simulink model "GPCA_Alarm"  (Simulink 8.7)
settings: Solver=VariableStepAuto  StartTime=0.0  StopTime=10.0  RelTol=1e-3
libraries: simulink x14
(part 2 of 3)

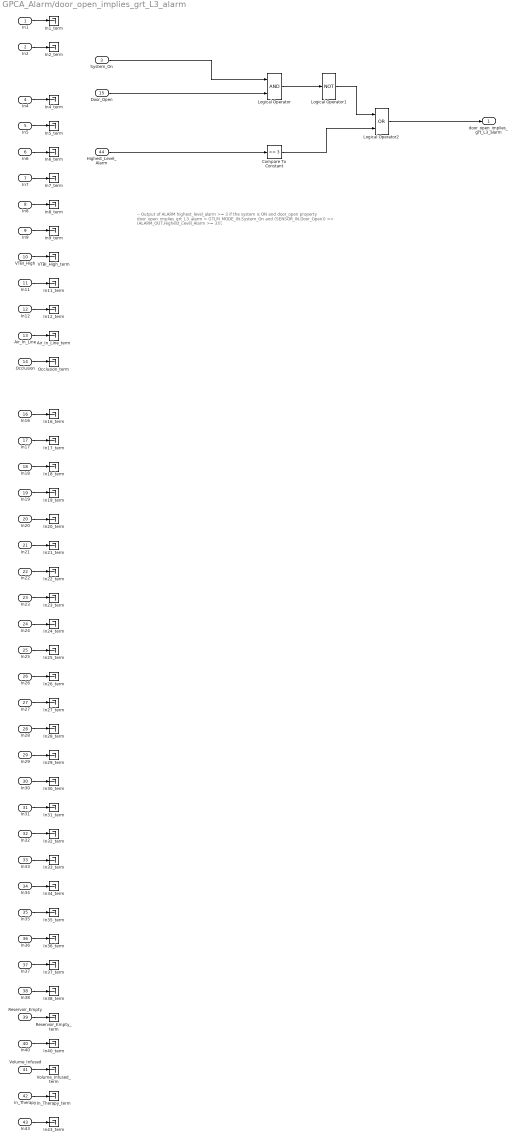
== system GPCA_Alarm/door_open_implies_grt_L3_alarm ==
  note: -- Output of ALARM highest_level_alarm >= 3 if the system is ON and door_open
      | property door_open_implies_grt_L3_alarm =
      | ((TLM_MODE_IN.System_On and (SENSOR_IN.Door_Open)) => (ALARM_OUT.Highest_Level_Alarm >= 3));
  In1 : Inport
  In2 : Inport  Port=2
  System_On : Inport  Port=3
  In4 : Inport  Port=4
  In5 : Inport  Port=5
  In6 : Inport  Port=6
  In7 : Inport  Port=7
  In8 : Inport  Port=8
  In9 : Inport  Port=9
  VTBI_High : Inport  Port=10
  In11 : Inport  Port=11
  In12 : Inport  Port=12
  Air_In_Line : Inport  Port=13
  Occlusion : Inport  Port=14
  Door_Open : Inport  Port=15
  In16 : Inport  Port=16
  In17 : Inport  Port=17
  In18 : Inport  Port=18
  In19 : Inport  Port=19
  In20 : Inport  Port=20
  In21 : Inport  Port=21
  In22 : Inport  Port=22
  In23 : Inport  Port=23
  In24 : Inport  Port=24
  In25 : Inport  Port=25
  In26 : Inport  Port=26
  In27 : Inport  Port=27
  In28 : Inport  Port=28
  In29 : Inport  Port=29
  In30 : Inport  Port=30
  In31 : Inport  Port=31
  In32 : Inport  Port=32
  In33 : Inport  Port=33
  In34 : Inport  Port=34
  In35 : Inport  Port=35
  In36 : Inport  Port=36
  In37 : Inport  Port=37
  In38 : Inport  Port=38
  Reservoir_Empty : Inport  Port=39
  In40 : Inport  Port=40
  Volume_Infused : Inport  Port=41
  In_Therapy : Inport  Port=42
  In43 : Inport  Port=43
  Highest_Level_Alarm : Inport  Port=44
  Air_In_Line_term : Terminator
  Compare To Constant : simulink/Logic and Bit Operations/Compare To Constant  relop=>=  const=3  OutDataTypeStr=boolean
  In11_term : Terminator
  In12_term : Terminator
  In16_term : Terminator
  In17_term : Terminator
  In18_term : Terminator
  In19_term : Terminator
  In1_term : Terminator
  In20_term : Terminator
  In21_term : Terminator
  In22_term : Terminator
  In23_term : Terminator
  In24_term : Terminator
  In25_term : Terminator
  In26_term : Terminator
  In27_term : Terminator
  In28_term : Terminator
  In29_term : Terminator
  In2_term : Terminator
  In30_term : Terminator
  In31_term : Terminator
  In32_term : Terminator
  In33_term : Terminator
  In34_term : Terminator
  In35_term : Terminator
  In36_term : Terminator
  In37_term : Terminator
  In38_term : Terminator
  In40_term : Terminator
  In43_term : Terminator
  In4_term : Terminator
  In5_term : Terminator
  In6_term : Terminator
  In7_term : Terminator
  In8_term : Terminator
  In9_term : Terminator
  In_Therapy_term : Terminator
  Logical Operator : Logic  AllPortsSameDT=off  OutDataTypeStr=boolean
  Logical Operator1 : Logic  Operator=NOT  Inputs=3  AllPortsSameDT=off  OutDataTypeStr=boolean
  Logical Operator2 : Logic  Operator=OR  AllPortsSameDT=off  OutDataTypeStr=boolean
  Occlusion_term : Terminator
  Reservoir_Empty_term : Terminator
  VTBI_High_term : Terminator
  Volume_Infused_term : Terminator
  door_open_implies_grt_L3_alarm : Outport
  wires:
  In1/1 -> In1_term/1
  In2/1 -> In2_term/1
  In4/1 -> In4_term/1
  In5/1 -> In5_term/1
  In6/1 -> In6_term/1
  In7/1 -> In7_term/1
  In8/1 -> In8_term/1
  In9/1 -> In9_term/1
  VTBI_High/1 -> VTBI_High_term/1
  In11/1 -> In11_term/1
  In12/1 -> In12_term/1
  Air_In_Line/1 -> Air_In_Line_term/1
  Occlusion/1 -> Occlusion_term/1
  In16/1 -> In16_term/1
  In17/1 -> In17_term/1
  In18/1 -> In18_term/1
  In19/1 -> In19_term/1
  In20/1 -> In20_term/1
  In21/1 -> In21_term/1
  In22/1 -> In22_term/1
  In23/1 -> In23_term/1
  In24/1 -> In24_term/1
  In25/1 -> In25_term/1
  In26/1 -> In26_term/1
  In27/1 -> In27_term/1
  In28/1 -> In28_term/1
  In29/1 -> In29_term/1
  In30/1 -> In30_term/1
  In31/1 -> In31_term/1
  In32/1 -> In32_term/1
  In33/1 -> In33_term/1
  In34/1 -> In34_term/1
  In35/1 -> In35_term/1
  In36/1 -> In36_term/1
  In37/1 -> In37_term/1
  In38/1 -> In38_term/1
  Reservoir_Empty/1 -> Reservoir_Empty_term/1
  In40/1 -> In40_term/1
  Volume_Infused/1 -> Volume_Infused_term/1
  In_Therapy/1 -> In_Therapy_term/1
  In43/1 -> In43_term/1
  System_On/1 -> Logical Operator/1
  Door_Open/1 -> Logical Operator/2
  Highest_Level_Alarm/1 -> Compare To Constant/1
  Logical Operator/1 -> Logical Operator1/1
  Logical Operator1/1 -> Logical Operator2/1
  Compare To Constant/1 -> Logical Operator2/2
  Logical Operator2/1 -> door_open_implies_grt_L3_alarm/1

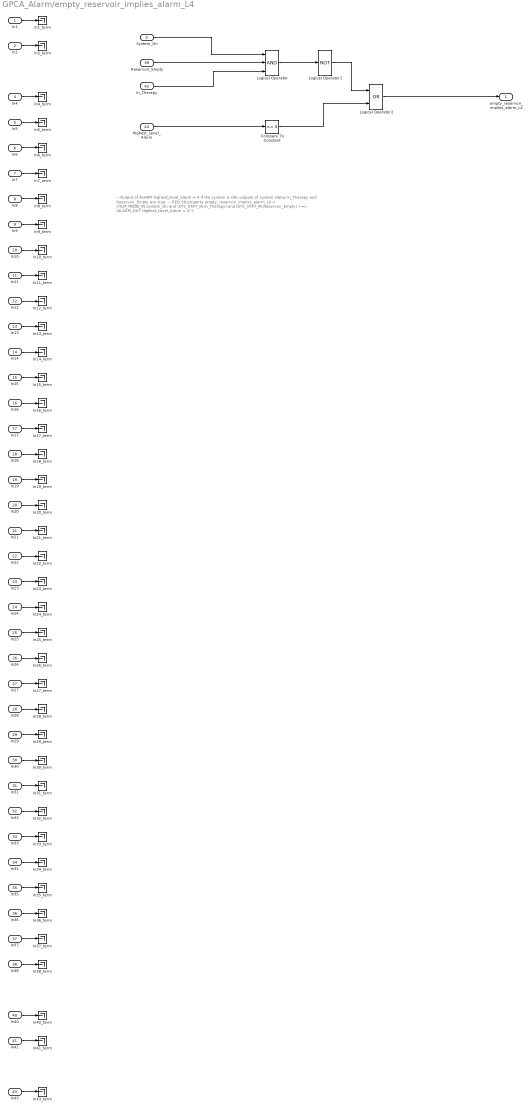
== system GPCA_Alarm/empty_reservoir_implies_alarm_L4 ==
  note: -- Output of ALARM highest_level_alarm = 4 if the system is ON, outputs of system status In_Therapy and Reservoir_Empty are true.
      | -- REQ 59
      | property empty_reservoir_implies_alarm_L4 =
      | ((TLM_MODE_IN.System_On and (SYS_STAT_IN.In_Therapy) and (SYS_STAT_IN.Reservoir_Empty) ) =>
      | (ALARM_OUT.Highest_Level_Alarm = 4) );
  In1 : Inport
  In2 : Inport  Port=2
  System_On : Inport  Port=3
  In4 : Inport  Port=4
  In5 : Inport  Port=5
  In6 : Inport  Port=6
  In7 : Inport  Port=7
  In8 : Inport  Port=8
  In9 : Inport  Port=9
  In10 : Inport  Port=10
  In11 : Inport  Port=11
  In12 : Inport  Port=12
  In13 : Inport  Port=13
  In14 : Inport  Port=14
  In15 : Inport  Port=15
  In16 : Inport  Port=16
  In17 : Inport  Port=17
  In18 : Inport  Port=18
  In19 : Inport  Port=19
  In20 : Inport  Port=20
  In21 : Inport  Port=21
  In22 : Inport  Port=22
  In23 : Inport  Port=23
  In24 : Inport  Port=24
  In25 : Inport  Port=25
  In26 : Inport  Port=26
  In27 : Inport  Port=27
  In28 : Inport  Port=28
  In29 : Inport  Port=29
  In30 : Inport  Port=30
  In31 : Inport  Port=31
  In32 : Inport  Port=32
  In33 : Inport  Port=33
  In34 : Inport  Port=34
  In35 : Inport  Port=35
  In36 : Inport  Port=36
  In37 : Inport  Port=37
  In38 : Inport  Port=38
  Reservoir_Empty : Inport  Port=39
  In40 : Inport  Port=40
  In41 : Inport  Port=41
  In_Therapy : Inport  Port=42
  In43 : Inport  Port=43
  Highest_Level_Alarm : Inport  Port=44
  Compare To Constant : simulink/Logic and Bit Operations/Compare To Constant  relop===  const=4  OutDataTypeStr=boolean
  In10_term : Terminator
  In11_term : Terminator
  In12_term : Terminator
  In13_term : Terminator
  In14_term : Terminator
  In15_term : Terminator
  In16_term : Terminator
  In17_term : Terminator
  In18_term : Terminator
  In19_term : Terminator
  In1_term : Terminator
  In20_term : Terminator
  In21_term : Terminator
  In22_term : Terminator
  In23_term : Terminator
  In24_term : Terminator
  In25_term : Terminator
  In26_term : Terminator
  In27_term : Terminator
  In28_term : Terminator
  In29_term : Terminator
  In2_term : Terminator
  In30_term : Terminator
  In31_term : Terminator
  In32_term : Terminator
  In33_term : Terminator
  In34_term : Terminator
  In35_term : Terminator
  In36_term : Terminator
  In37_term : Terminator
  In38_term : Terminator
  In40_term : Terminator
  In41_term : Terminator
  In43_term : Terminator
  In4_term : Terminator
  In5_term : Terminator
  In6_term : Terminator
  In7_term : Terminator
  In8_term : Terminator
  In9_term : Terminator
  Logical Operator : Logic  Inputs=3  AllPortsSameDT=off  OutDataTypeStr=boolean
  Logical Operator1 : Logic  Operator=NOT  Inputs=3  AllPortsSameDT=off  OutDataTypeStr=boolean
  Logical Operator2 : Logic  Operator=OR  AllPortsSameDT=off  OutDataTypeStr=boolean
  empty_reservoir_implies_alarm_L4 : Outport
  wires:
  In1/1 -> In1_term/1
  In2/1 -> In2_term/1
  System_On/1 -> Logical Operator/1
  In4/1 -> In4_term/1
  In5/1 -> In5_term/1
  In6/1 -> In6_term/1
  In7/1 -> In7_term/1
  In8/1 -> In8_term/1
  In9/1 -> In9_term/1
  In10/1 -> In10_term/1
  In11/1 -> In11_term/1
  In12/1 -> In12_term/1
  In13/1 -> In13_term/1
  In14/1 -> In14_term/1
  In15/1 -> In15_term/1
  In16/1 -> In16_term/1
  In17/1 -> In17_term/1
  In18/1 -> In18_term/1
  In19/1 -> In19_term/1
  In20/1 -> In20_term/1
  In21/1 -> In21_term/1
  In22/1 -> In22_term/1
  In23/1 -> In23_term/1
  In24/1 -> In24_term/1
  In25/1 -> In25_term/1
  In26/1 -> In26_term/1
  In27/1 -> In27_term/1
  In28/1 -> In28_term/1
  In29/1 -> In29_term/1
  In30/1 -> In30_term/1
  In31/1 -> In31_term/1
  In32/1 -> In32_term/1
  In33/1 -> In33_term/1
  In34/1 -> In34_term/1
  In35/1 -> In35_term/1
  In36/1 -> In36_term/1
  In37/1 -> In37_term/1
  In38/1 -> In38_term/1
  Reservoir_Empty/1 -> Logical Operator/2
  In40/1 -> In40_term/1
  In41/1 -> In41_term/1
  In_Therapy/1 -> Logical Operator/3
  In43/1 -> In43_term/1
  Highest_Level_Alarm/1 -> Compare To Constant/1
  Logical Operator/1 -> Logical Operator1/1
  Logical Operator1/1 -> Logical Operator2/1
  Compare To Constant/1 -> Logical Operator2/2
  Logical Operator2/1 -> empty_reservoir_implies_alarm_L4/1

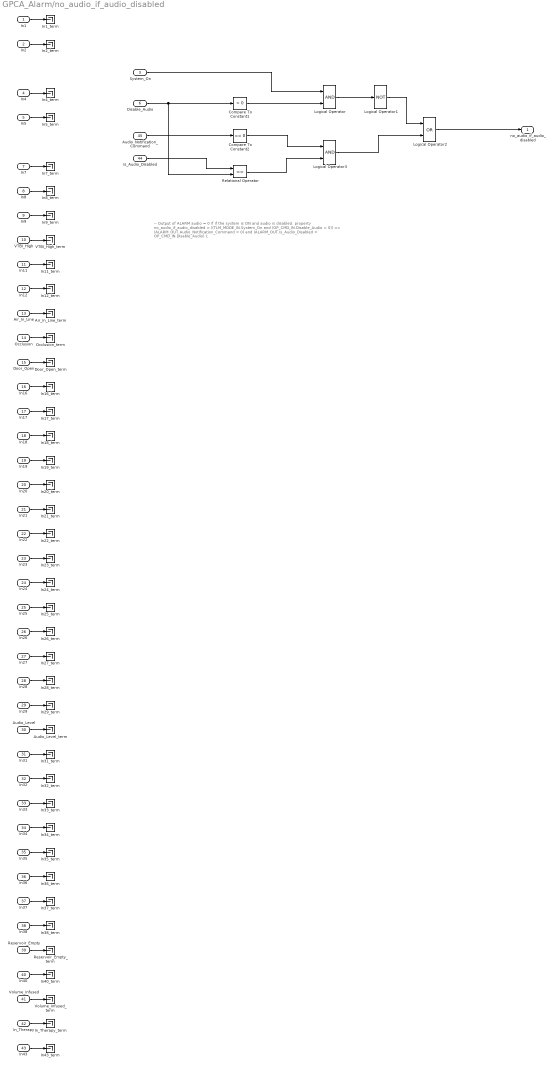
== system GPCA_Alarm/no_audio_if_audio_disabled ==
  note: -- Output of ALARM audio = 0 if if the system is ON and audio is disabled.
      | property no_audio_if_audio_disabled =
      | ((TLM_MODE_IN.System_On and (OP_CMD_IN.Disable_Audio > 0))
      | => (ALARM_OUT.Audio_Notification_Command = 0) and (ALARM_OUT.Is_Audio_Disabled = OP_CMD_IN.Disable_Audio) );
  In1 : Inport
  In2 : Inport  Port=2
  System_On : Inport  Port=3
  In4 : Inport  Port=4
  In5 : Inport  Port=5
  Disable_Audio : Inport  Port=6
  In7 : Inport  Port=7
  In8 : Inport  Port=8
  In9 : Inport  Port=9
  VTBI_High : Inport  Port=10
  In11 : Inport  Port=11
  In12 : Inport  Port=12
  Air_In_Line : Inport  Port=13
  Occlusion : Inport  Port=14
  Door_Open : Inport  Port=15
  In16 : Inport  Port=16
  In17 : Inport  Port=17
  In18 : Inport  Port=18
  In19 : Inport  Port=19
  In20 : Inport  Port=20
  In21 : Inport  Port=21
  In22 : Inport  Port=22
  In23 : Inport  Port=23
  In24 : Inport  Port=24
  In25 : Inport  Port=25
  In26 : Inport  Port=26
  In27 : Inport  Port=27
  In28 : Inport  Port=28
  In29 : Inport  Port=29
  Audio_Level : Inport  Port=30
  In31 : Inport  Port=31
  In32 : Inport  Port=32
  In33 : Inport  Port=33
  In34 : Inport  Port=34
  In35 : Inport  Port=35
  In36 : Inport  Port=36
  In37 : Inport  Port=37
  In38 : Inport  Port=38
  Reservoir_Empty : Inport  Port=39
  In40 : Inport  Port=40
  Volume_Infused : Inport  Port=41
  In_Therapy : Inport  Port=42
  In43 : Inport  Port=43
  Is_Audio_Disabled : Inport  Port=44
  Audio_Notification_Command : Inport  Port=45
  Air_In_Line_term : Terminator
  Audio_Level_term : Terminator
  Compare To Constant1 : simulink/Logic and Bit Operations/Compare To Constant  relop=>  const=0  OutDataTypeStr=boolean
  Compare To Constant2 : simulink/Logic and Bit Operations/Compare To Constant  relop===  const=0  OutDataTypeStr=boolean
  Door_Open_term : Terminator
  In11_term : Terminator
  In12_term : Terminator
  In16_term : Terminator
  In17_term : Terminator
  In18_term : Terminator
  In19_term : Terminator
  In1_term : Terminator
  In20_term : Terminator
  In21_term : Terminator
  In22_term : Terminator
  In23_term : Terminator
  In24_term : Terminator
  In25_term : Terminator
  In26_term : Terminator
  In27_term : Terminator
  In28_term : Terminator
  In29_term : Terminator
  In2_term : Terminator
  In31_term : Terminator
  In32_term : Terminator
  In33_term : Terminator
  In34_term : Terminator
  In35_term : Terminator
  In36_term : Terminator
  In37_term : Terminator
  In38_term : Terminator
  In40_term : Terminator
  In43_term : Terminator
  In4_term : Terminator
  In5_term : Terminator
  In7_term : Terminator
  In8_term : Terminator
  In9_term : Terminator
  In_Therapy_term : Terminator
  Logical Operator : Logic  AllPortsSameDT=off  OutDataTypeStr=boolean
  Logical Operator1 : Logic  Operator=NOT  Inputs=3  AllPortsSameDT=off  OutDataTypeStr=boolean
  Logical Operator2 : Logic  Operator=OR  AllPortsSameDT=off  OutDataTypeStr=boolean
  Logical Operator3 : Logic  AllPortsSameDT=off  OutDataTypeStr=boolean
  Occlusion_term : Terminator
  Relational Operator : RelationalOperator  Operator===  OutDataTypeStr=boolean
  Reservoir_Empty_term : Terminator
  VTBI_High_term : Terminator
  Volume_Infused_term : Terminator
  no_audio_if_audio_disabled : Outport
  wires:
  In1/1 -> In1_term/1
  In2/1 -> In2_term/1
  In4/1 -> In4_term/1
  In5/1 -> In5_term/1
  In7/1 -> In7_term/1
  In8/1 -> In8_term/1
  In9/1 -> In9_term/1
  VTBI_High/1 -> VTBI_High_term/1
  In11/1 -> In11_term/1
  In12/1 -> In12_term/1
  Air_In_Line/1 -> Air_In_Line_term/1
  Occlusion/1 -> Occlusion_term/1
  Door_Open/1 -> Door_Open_term/1
  In16/1 -> In16_term/1
  In17/1 -> In17_term/1
  In18/1 -> In18_term/1
  In19/1 -> In19_term/1
  In20/1 -> In20_term/1
  In21/1 -> In21_term/1
  In22/1 -> In22_term/1
  In23/1 -> In23_term/1
  In24/1 -> In24_term/1
  In25/1 -> In25_term/1
  In26/1 -> In26_term/1
  In27/1 -> In27_term/1
  In28/1 -> In28_term/1
  In29/1 -> In29_term/1
  Audio_Level/1 -> Audio_Level_term/1
  In31/1 -> In31_term/1
  In32/1 -> In32_term/1
  In33/1 -> In33_term/1
  In34/1 -> In34_term/1
  In35/1 -> In35_term/1
  In36/1 -> In36_term/1
  In37/1 -> In37_term/1
  In38/1 -> In38_term/1
  Reservoir_Empty/1 -> Reservoir_Empty_term/1
  In40/1 -> In40_term/1
  Volume_Infused/1 -> Volume_Infused_term/1
  In_Therapy/1 -> In_Therapy_term/1
  In43/1 -> In43_term/1
  Audio_Notification_Command/1 -> Compare To Constant2/1
  Disable_Audio/1 -> Relational Operator/2, Compare To Constant1/1
  Is_Audio_Disabled/1 -> Relational Operator/1
  System_On/1 -> Logical Operator/1
  Logical Operator/1 -> Logical Operator1/1
  Logical Operator1/1 -> Logical Operator2/1
  Logical Operator2/1 -> no_audio_if_audio_disabled/1
  Compare To Constant1/1 -> Logical Operator/2
  Compare To Constant2/1 -> Logical Operator3/1
  Relational Operator/1 -> Logical Operator3/2
  Logical Operator3/1 -> Logical Operator2/2

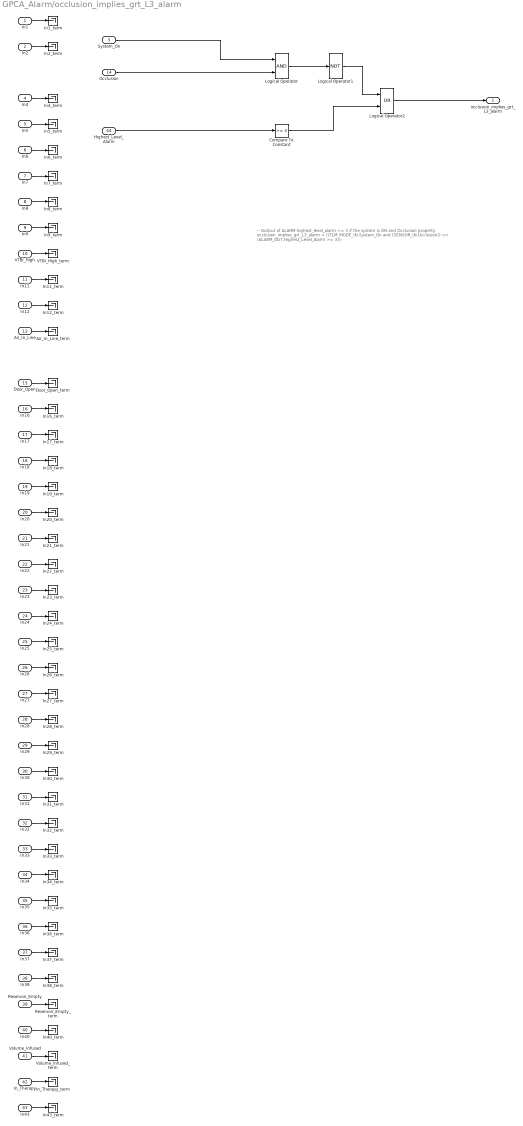
== system GPCA_Alarm/occlusion_implies_grt_L3_alarm ==
  note: -- Output of ALARM highest_level_alarm >= 3 if the system is ON and Occlusion
      | property occlusion_implies_grt_L3_alarm =
      | ((TLM_MODE_IN.System_On and (SENSOR_IN.Occlusion)) => (ALARM_OUT.Highest_Level_Alarm >= 3));
  In1 : Inport
  In2 : Inport  Port=2
  System_On : Inport  Port=3
  In4 : Inport  Port=4
  In5 : Inport  Port=5
  In6 : Inport  Port=6
  In7 : Inport  Port=7
  In8 : Inport  Port=8
  In9 : Inport  Port=9
  VTBI_High : Inport  Port=10
  In11 : Inport  Port=11
  In12 : Inport  Port=12
  Air_In_Line : Inport  Port=13
  Occlusion : Inport  Port=14
  Door_Open : Inport  Port=15
  In16 : Inport  Port=16
  In17 : Inport  Port=17
  In18 : Inport  Port=18
  In19 : Inport  Port=19
  In20 : Inport  Port=20
  In21 : Inport  Port=21
  In22 : Inport  Port=22
  In23 : Inport  Port=23
  In24 : Inport  Port=24
  In25 : Inport  Port=25
  In26 : Inport  Port=26
  In27 : Inport  Port=27
  In28 : Inport  Port=28
  In29 : Inport  Port=29
  In30 : Inport  Port=30
  In31 : Inport  Port=31
  In32 : Inport  Port=32
  In33 : Inport  Port=33
  In34 : Inport  Port=34
  In35 : Inport  Port=35
  In36 : Inport  Port=36
  In37 : Inport  Port=37
  In38 : Inport  Port=38
  Reservoir_Empty : Inport  Port=39
  In40 : Inport  Port=40
  Volume_Infused : Inport  Port=41
  In_Therapy : Inport  Port=42
  In43 : Inport  Port=43
  Highest_Level_Alarm : Inport  Port=44
  Air_In_Line_term : Terminator
  Compare To Constant : simulink/Logic and Bit Operations/Compare To Constant  relop=>=  const=3  OutDataTypeStr=boolean
  Door_Open_term : Terminator
  In11_term : Terminator
  In12_term : Terminator
  In16_term : Terminator
  In17_term : Terminator
  In18_term : Terminator
  In19_term : Terminator
  In1_term : Terminator
  In20_term : Terminator
  In21_term : Terminator
  In22_term : Terminator
  In23_term : Terminator
  In24_term : Terminator
  In25_term : Terminator
  In26_term : Terminator
  In27_term : Terminator
  In28_term : Terminator
  In29_term : Terminator
  In2_term : Terminator
  In30_term : Terminator
  In31_term : Terminator
  In32_term : Terminator
  In33_term : Terminator
  In34_term : Terminator
  In35_term : Terminator
  In36_term : Terminator
  In37_term : Terminator
  In38_term : Terminator
  In40_term : Terminator
  In43_term : Terminator
  In4_term : Terminator
  In5_term : Terminator
  In6_term : Terminator
  In7_term : Terminator
  In8_term : Terminator
  In9_term : Terminator
  In_Therapy_term : Terminator
  Logical Operator : Logic  AllPortsSameDT=off  OutDataTypeStr=boolean
  Logical Operator1 : Logic  Operator=NOT  Inputs=3  AllPortsSameDT=off  OutDataTypeStr=boolean
  Logical Operator2 : Logic  Operator=OR  AllPortsSameDT=off  OutDataTypeStr=boolean
  Reservoir_Empty_term : Terminator
  VTBI_High_term : Terminator
  Volume_Infused_term : Terminator
  occlusion_implies_grt_L3_alarm : Outport
  wires:
  In1/1 -> In1_term/1
  In2/1 -> In2_term/1
  In4/1 -> In4_term/1
  In5/1 -> In5_term/1
  In6/1 -> In6_term/1
  In7/1 -> In7_term/1
  In8/1 -> In8_term/1
  In9/1 -> In9_term/1
  VTBI_High/1 -> VTBI_High_term/1
  In11/1 -> In11_term/1
  In12/1 -> In12_term/1
  Air_In_Line/1 -> Air_In_Line_term/1
  Door_Open/1 -> Door_Open_term/1
  In16/1 -> In16_term/1
  In17/1 -> In17_term/1
  In18/1 -> In18_term/1
  In19/1 -> In19_term/1
  In20/1 -> In20_term/1
  In21/1 -> In21_term/1
  In22/1 -> In22_term/1
  In23/1 -> In23_term/1
  In24/1 -> In24_term/1
  In25/1 -> In25_term/1
  In26/1 -> In26_term/1
  In27/1 -> In27_term/1
  In28/1 -> In28_term/1
  In29/1 -> In29_term/1
  In30/1 -> In30_term/1
  In31/1 -> In31_term/1
  In32/1 -> In32_term/1
  In33/1 -> In33_term/1
  In34/1 -> In34_term/1
  In35/1 -> In35_term/1
  In36/1 -> In36_term/1
  In37/1 -> In37_term/1
  In38/1 -> In38_term/1
  Reservoir_Empty/1 -> Reservoir_Empty_term/1
  In40/1 -> In40_term/1
  Volume_Infused/1 -> Volume_Infused_term/1
  In_Therapy/1 -> In_Therapy_term/1
  In43/1 -> In43_term/1
  System_On/1 -> Logical Operator/1
  Occlusion/1 -> Logical Operator/2
  Highest_Level_Alarm/1 -> Compare To Constant/1
  Logical Operator/1 -> Logical Operator1/1
  Logical Operator1/1 -> Logical Operator2/1
  Compare To Constant/1 -> Logical Operator2/2
  Logical Operator2/1 -> occlusion_implies_grt_L3_alarm/1

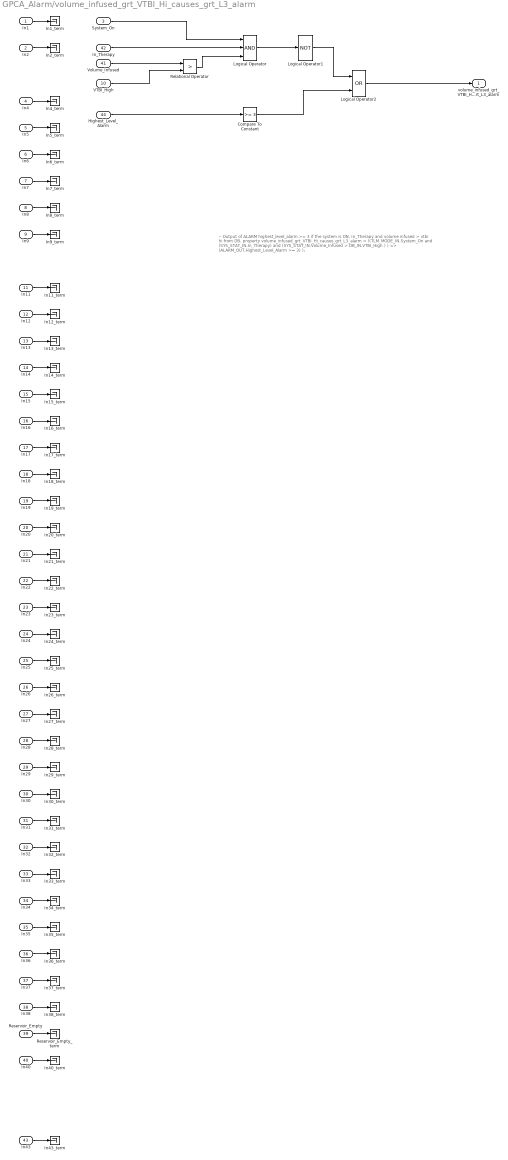
== system GPCA_Alarm/volume_infused_grt_VTBI_Hi_causes_grt_L3_alarm ==
  note: -- Output of ALARM highest_level_alarm >= 3 if the system is ON, In_Therapy and volume infused > vtbi hi from DB.
      | property volume_infused_grt_VTBI_Hi_causes_grt_L3_alarm =
      | ((TLM_MODE_IN.System_On and (SYS_STAT_IN.In_Therapy) and (SYS_STAT_IN.Volume_Infused > DB_IN.VTBI_High ) ) =>
      | (ALARM_OUT.Highest_Level_Alarm >= 3) );
  In1 : Inport
  In2 : Inport  Port=2
  System_On : Inport  Port=3
  In4 : Inport  Port=4
  In5 : Inport  Port=5
  In6 : Inport  Port=6
  In7 : Inport  Port=7
  In8 : Inport  Port=8
  In9 : Inport  Port=9
  VTBI_High : Inport  Port=10
  In11 : Inport  Port=11
  In12 : Inport  Port=12
  In13 : Inport  Port=13
  In14 : Inport  Port=14
  In15 : Inport  Port=15
  In16 : Inport  Port=16
  In17 : Inport  Port=17
  In18 : Inport  Port=18
  In19 : Inport  Port=19
  In20 : Inport  Port=20
  In21 : Inport  Port=21
  In22 : Inport  Port=22
  In23 : Inport  Port=23
  In24 : Inport  Port=24
  In25 : Inport  Port=25
  In26 : Inport  Port=26
  In27 : Inport  Port=27
  In28 : Inport  Port=28
  In29 : Inport  Port=29
  In30 : Inport  Port=30
  In31 : Inport  Port=31
  In32 : Inport  Port=32
  In33 : Inport  Port=33
  In34 : Inport  Port=34
  In35 : Inport  Port=35
  In36 : Inport  Port=36
  In37 : Inport  Port=37
  In38 : Inport  Port=38
  Reservoir_Empty : Inport  Port=39
  In40 : Inport  Port=40
  Volume_Infused : Inport  Port=41
  In_Therapy : Inport  Port=42
  In43 : Inport  Port=43
  Highest_Level_Alarm : Inport  Port=44
  Compare To Constant : simulink/Logic and Bit Operations/Compare To Constant  relop=>=  const=3  OutDataTypeStr=boolean
  In11_term : Terminator
  In12_term : Terminator
  In13_term : Terminator
  In14_term : Terminator
  In15_term : Terminator
  In16_term : Terminator
  In17_term : Terminator
  In18_term : Terminator
  In19_term : Terminator
  In1_term : Terminator
  In20_term : Terminator
  In21_term : Terminator
  In22_term : Terminator
  In23_term : Terminator
  In24_term : Terminator
  In25_term : Terminator
  In26_term : Terminator
  In27_term : Terminator
  In28_term : Terminator
  In29_term : Terminator
  In2_term : Terminator
  In30_term : Terminator
  In31_term : Terminator
  In32_term : Terminator
  In33_term : Terminator
  In34_term : Terminator
  In35_term : Terminator
  In36_term : Terminator
  In37_term : Terminator
  In38_term : Terminator
  In40_term : Terminator
  In43_term : Terminator
  In4_term : Terminator
  In5_term : Terminator
  In6_term : Terminator
  In7_term : Terminator
  In8_term : Terminator
  In9_term : Terminator
  Logical Operator : Logic  Inputs=3  AllPortsSameDT=off  OutDataTypeStr=boolean
  Logical Operator1 : Logic  Operator=NOT  Inputs=3  AllPortsSameDT=off  OutDataTypeStr=boolean
  Logical Operator2 : Logic  Operator=OR  AllPortsSameDT=off  OutDataTypeStr=boolean
  Relational Operator : RelationalOperator  Operator=>  OutDataTypeStr=boolean
  Reservoir_Empty_term : Terminator
  volume_infused_grt_VTBI_Hi_causes_grt_L3_alarm : Outport
  wires:
  In1/1 -> In1_term/1
  In2/1 -> In2_term/1
  In4/1 -> In4_term/1
  In5/1 -> In5_term/1
  In6/1 -> In6_term/1
  In7/1 -> In7_term/1
  In8/1 -> In8_term/1
  In9/1 -> In9_term/1
  VTBI_High/1 -> Relational Operator/2
  In11/1 -> In11_term/1
  In12/1 -> In12_term/1
  In13/1 -> In13_term/1
  In14/1 -> In14_term/1
  In15/1 -> In15_term/1
  In16/1 -> In16_term/1
  In17/1 -> In17_term/1
  In18/1 -> In18_term/1
  In19/1 -> In19_term/1
  In20/1 -> In20_term/1
  In21/1 -> In21_term/1
  In22/1 -> In22_term/1
  In23/1 -> In23_term/1
  In24/1 -> In24_term/1
  In25/1 -> In25_term/1
  In26/1 -> In26_term/1
  In27/1 -> In27_term/1
  In28/1 -> In28_term/1
  In29/1 -> In29_term/1
  In30/1 -> In30_term/1
  In31/1 -> In31_term/1
  In32/1 -> In32_term/1
  In33/1 -> In33_term/1
  In34/1 -> In34_term/1
  In35/1 -> In35_term/1
  In36/1 -> In36_term/1
  In37/1 -> In37_term/1
  In38/1 -> In38_term/1
  Reservoir_Empty/1 -> Reservoir_Empty_term/1
  In40/1 -> In40_term/1
  Volume_Infused/1 -> Relational Operator/1
  In43/1 -> In43_term/1
  System_On/1 -> Logical Operator/1
  In_Therapy/1 -> Logical Operator/2
  Relational Operator/1 -> Logical Operator/3
  Highest_Level_Alarm/1 -> Compare To Constant/1
  Logical Operator/1 -> Logical Operator1/1
  Logical Operator1/1 -> Logical Operator2/1
  Compare To Constant/1 -> Logical Operator2/2
  Logical Operator2/1 -> volume_infused_grt_VTBI_Hi_causes_grt_L3_alarm/1
